simulink model "F3_CAN_LoopBackInterrupt"  (R2018b)
settings: Solver=FixedStepDiscrete  StartTime=0.0  StopTime=10.0  RelTol=1e-3  EnableMultiTasking=on
libraries: CAN_Lib x13, canmsglib x2, STM32_Config_Lib x1
settings Model: Creator=reynaudp  LastModifiedBy=fenard1
settings DataIOCC: LimitDataPoints=on  SaveFormat=Array
settings OptimizationCC: DefaultParameterBehavior=Inlined  DefaultUnderspecifiedDataType=single  PassReuseOutputArgsAs=Individual arguments  LifeSpan=1
settings DebuggingCC: SolverPrmCheckMsg=warning  UniqueDataStoreMsg=error  AllowSymbolicDim=off  StrictBusMsg=ErrorOnBusTreatedAsVector  SFUnexpectedBacktrackingDiag=warning  SFNoUnconditionalDefaultTransitionDiag=warning  SFUndirectedBroadcastEventsDiag=error  SFExecutionAtInitializationDiag=none
settings HardwareCC: ProdBitPerPointer=32  ProdBitPerSizeT=32  ProdBitPerPtrDiffT=32  ProdLargestAtomicInteger=Integer  ProdWordSize=32  ProdHWDeviceType=STMicroelectronics->STM32 32-bit Cortex-M
settings ModelReferenceCC: PropagateSignalLabelsOutOfModel=off
settings SFSimCC: SimUseLocalCustomCode=off  CompileTimeRecursionLimit=0  EnableRuntimeRecursion=off  MATLABDynamicMemAlloc=off
settings RTWCC: SystemTargetFile=stm32.tlc  TemplateMakefile=stm32.tmf  Description=stm32 (Embedded Target)  GenerateReport=on  RTWUseLocalCustomCode=off  Toolchain=Microsoft Windows SDK v7.1 | nmake (64-bit Windows)
settings CodeAppCC: IgnoreCustomStorageClasses=off  CustomSymbolStrType=$N$R$M  SimulinkBlockComments=off
settings STFCustomTargetCC: TargetLangStandard=C99 (ISO)  ParMdlRefBuildCompliant=on  IncludeMdlTerminateFcn=off  CombineOutputUpdateFcns=on  ERTCustomFileBanners=on  SupportComplex=off  SupportContinuousTime=off  SupportNonInlinedSFcns=off  RemoveResetFunc=on  ParenthesesLevel=Maximum  CastingMode=Standards  MATLABClassNameForMDSCustomization=Simulink.SoftwareTarget.ERTCustomization  SystemTargetFile=stm32.tlc
settings ERTTargetCC: TargetLangStandard=C99 (ISO)  MultiwordLength=2048  CompOptLevelCompliant=off  ConcurrentExecutionCompliant=off  IncludeMdlTerminateFcn=off  SupportComplex=off  ParenthesesLevel=Maximum  CastingMode=Standards  ModelStepFunctionPrototypeControlCompliant=off  CPPClassGenCompliant=off  UseToolchainInfoCompliant=off  ERTSrcFileBannerTemplate=sourceFileTemplate.cgt  ERTHdrFileBannerTemplate=sourceFileTemplate.cgt  ERTDataSrcFileTemplate=sourceFileTemplate.cgt  ERTDataHdrFileTemplate=sourceFileTemplate.cgt  ERTCustomFileTemplate=customRoutineProcess.tlc  ConvertIfToSwitch=off  SuppressUnreachableDefaultCases=off  EnableSignedLeftShifts=off  EnableSignedRightShifts=off
settings ConfigComp: CovMetricSettings=dw  CovHtmlReporting=on  CovSaveCumulativeToWorkspaceVar=on  CovSaveSingleToWorkspaceVar=on  CovExternalEMLEnable=off  CovSFcnEnable=off

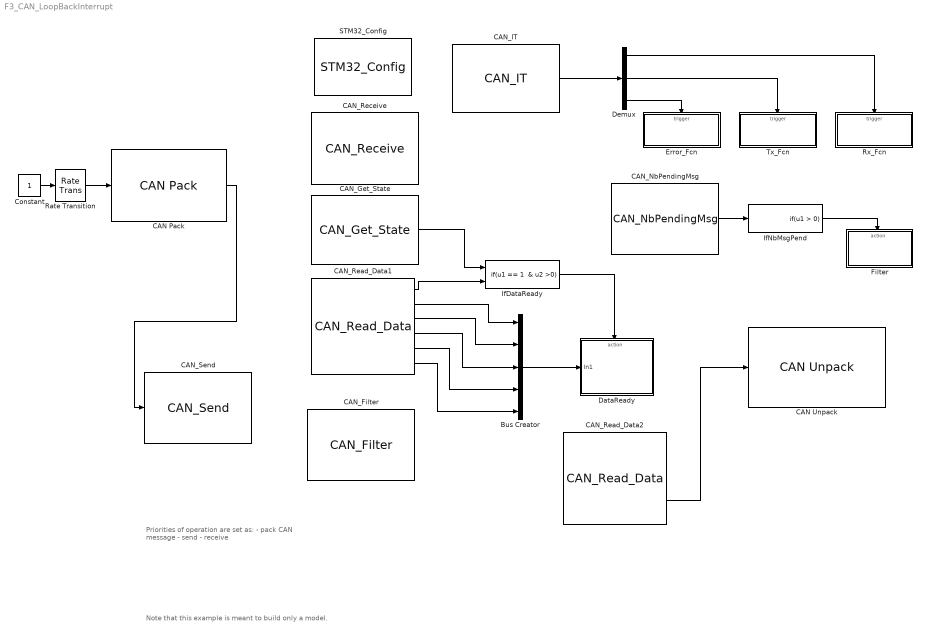
== system F3_CAN_LoopBackInterrupt ==
  note: Priorities of operation are set as:
      | - pack CAN message
      | - send
      | - receive
  note: Note that this example is meant to build only a model.
  Bus Creator : BusCreator  Inputs=5
  CAN Pack : canmsglib/CAN Pack  Priority=1  MsgList=(none)  MsgName=CAN Msg  MsgIDType=Extended (29-bit identifier)  MsgIdentifier=0  MsgLength=8  SignalInfo=Signal1$0$8$1$1$1$0$1$0$-Inf$Inf$#  NSignals=1  StartBits=str2num('[int32(0)]')  SignalSizes=str2num('[int32(8)]')  ByteOrders=str2num('[int32(1)]')  DataTypes=str2num('[int32(1)]')  MultiplexTypes=str2num('[int32(1)]')  MultiplexValues=str2num('[double(0)]')  Factors=str2num('[double(1)]')  Offsets=str2num('[double(0)]')  Minimums=str2num('[double(-Inf)]')  Maximums=str2num('[double(Inf)]')  Remote=off  ApplyMinMax=off  BusOutput=off
      settings: AttributesFormatString=Priority=%<Priority>  SourceProductName=Vehicle Network Toolbox  SourceProductBaseCode=VN  DataFormat=manually specified signals
  CAN Unpack : canmsglib/CAN Unpack  MsgList=(none)  MsgName=CAN Msg  MsgIDType=Standard (11-bit identifier)  MsgIdentifier=0  MsgLength=8  NSignals=0  IDPort=on  TimestampPort=on  ErrorPort=on  RemotePort=on  LengthPort=on  StatusPort=on  StartBits=0  SignalSizes=0  ByteOrders=0  DataTypes=0  MultiplexTypes=0  MultiplexValues=0  Factors=0  Offsets=0  Minimums=0  Maximums=0  ApplyMinMax=off
      settings: SourceProductName=Vehicle Network Toolbox  SourceProductBaseCode=VN  DataFormat=raw data
  CAN_Filter : CAN_Lib/CAN_Filter  CAN_name=CAN  CAN_Filter_Activation=on  CAN_Filter_Scale=CAN_FILTERSCALE_32BIT  CAN_Filter_Mask_Id_High=0  CAN_Filter_Mask_Id_Low=0  CAN_Filter_Id_High=0  CAN_Filter_Id_Low=0  CAN_Filter_FIFO_Assignment=CAN_FIFO0  CAN_Filter_Bank=0  CAN_Filter_Mode=CAN_FILTERMODE_IDMASK  CAN_Filter_Slave_Start_Bank=14
      settings: SourceProductName=Target Support Package - STM32 Adapter
  CAN_Get_State : CAN_Lib/CAN_Get_State  CAN_name=CAN
      settings: SourceProductName=Target Support Package - STM32 Adapter
  CAN_IT : CAN_Lib/CAN_IT  CAN_name=CAN  CAN_Mode=Master  CAN_It=on  CAN_RX_It=on  CAN_TX_It=on  CAN_ERROR_It=on
      settings: SourceProductName=Target Support Package - STM32 Adapter
  CAN_NbPendingMsg : CAN_Lib/CAN_NbPendingMsg  CAN_name=CAN  CAN_Mode=Master  CAN_It=on  CAN_Fifo=CAN_FIFO0
      settings: SourceProductName=Target Support Package - STM32 Adapter
  CAN_Read_Data1 : CAN_Lib/CAN_Read_Data  CAN_name=CAN  CAN_Fifo=CAN_FIFO0  CAN_MsgType=off
      settings: SourceProductName=Target Support Package - STM32 Adapter
  CAN_Read_Data2 : CAN_Lib/CAN_Read_Data  CAN_name=CAN  CAN_Fifo=CAN_FIFO0  CAN_MsgType=on
      settings: SourceProductName=Target Support Package - STM32 Adapter
  CAN_Receive : CAN_Lib/CAN_Receive  Priority=2  CAN_name=CAN  CAN_Mode=Master  CAN_It=on  CAN_Fifo=CAN_FIFO0
      settings: AttributesFormatString=Priority=%<Priority>  SourceProductName=Target Support Package - STM32 Adapter
  CAN_Send : CAN_Lib/CAN_Send  Priority=2  CAN_name=CAN  CAN_Mode=Master  CAN_It=on  CAN_MsgType=on
      settings: AttributesFormatString=Priority=%<Priority>  SourceProductName=Target Support Package - STM32 Adapter
  Constant : Constant
  DataReady : Subsystem  TreatAsAtomicUnit=on
  Demux : Demux  Outputs=3
  Error_Fcn : Subsystem  TreatAsAtomicUnit=on
  Filter : Subsystem  TreatAsAtomicUnit=on
  IfDataReady : If  NumInputs=2  IfExpression="u1 == 1  & u2 >0"  ShowElse=off
  IfNbMsgPend : If  ShowElse=off
  Rate Transition : RateTransition
  Rx_Fcn : Subsystem  TreatAsAtomicUnit=on
  STM32_Config : STM32_Config_Lib/STM32_Config  Priority=0  Project_Path=.\  Config_File=F3_CAN_LoopBackInterrupt.ioc  MCU_Name=STM32F302R8Tx
      settings: SourceProductName=Target Support Package - STM32 Adapter
  Tx_Fcn : Subsystem  TreatAsAtomicUnit=on
  wires:
  CAN_IT/1 -> Demux/1
  Demux/1 -> Rx_Fcn/Trigger
  Demux/2 -> Tx_Fcn/Trigger
  Demux/3 -> Error_Fcn/Trigger
  IfDataReady/1 -> DataReady/Action
  CAN_Read_Data1/2 -> Bus Creator/1
  CAN_Read_Data1/3 -> Bus Creator/2
  CAN_Read_Data1/4 -> Bus Creator/3
  Bus Creator/1 -> DataReady/1(In1)
  CAN_Get_State/1 -> IfDataReady/1
  CAN_NbPendingMsg/1 -> IfNbMsgPend/1
  IfNbMsgPend/1 -> Filter/Action
  CAN_Read_Data1/1 -> IfDataReady/2
  CAN_Read_Data2/2 -> CAN Unpack/1
  CAN_Read_Data1/5 -> Bus Creator/4
  CAN_Read_Data1/6 -> Bus Creator/5
  CAN Pack/1 -> CAN_Send/1
  Constant/1 -> Rate Transition/1
  Rate Transition/1 -> CAN Pack/1

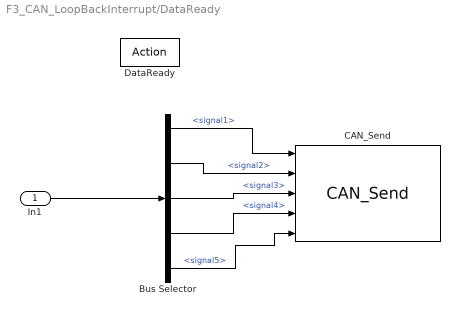
== system F3_CAN_LoopBackInterrupt/DataReady ==
  In1 : Inport
  DataReady : ActionPort  ActionType=then
  Bus Selector : BusSelector  OutputSignals=signal1,signal2,signal3,signal4,signal5
  CAN_Send : CAN_Lib/CAN_Send  CAN_name=CAN  CAN_Mode=Master  CAN_It=on  CAN_MsgType=off
      settings: SourceProductName=Target Support Package - STM32 Adapter
  wires:
  In1/1 -> Bus Selector/1
  Bus Selector/2 -> CAN_Send/2  "<signal2>"
  Bus Selector/3 -> CAN_Send/3  "<signal3>"
  Bus Selector/4 -> CAN_Send/4  "<signal4>"
  Bus Selector/5 -> CAN_Send/5  "<signal5>"
  Bus Selector/1 -> CAN_Send/1  "<signal1>"

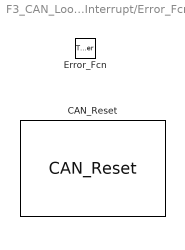
== system F3_CAN_LoopBackInterrupt/Error_Fcn ==
  Error_Fcn : TriggerPort  TriggerType=function-call  VariantControl=Variant
  CAN_Reset : CAN_Lib/CAN_Reset  CAN_name=CAN
      settings: SourceProductName=Target Support Package - STM32 Adapter

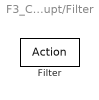
== system F3_CAN_LoopBackInterrupt/Filter ==
  Filter : ActionPort  ActionType=then

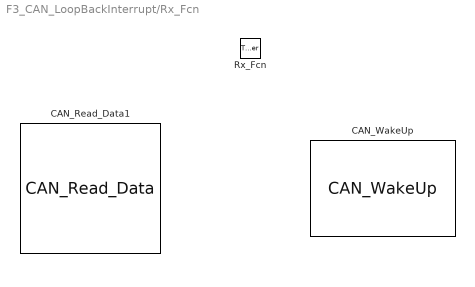
== system F3_CAN_LoopBackInterrupt/Rx_Fcn ==
  Rx_Fcn : TriggerPort  TriggerType=function-call  VariantControl=Variant
  CAN_Read_Data1 : CAN_Lib/CAN_Read_Data  CAN_name=CAN  CAN_Fifo=CAN_FIFO0  CAN_MsgType=off
      settings: SourceProductName=Target Support Package - STM32 Adapter
  CAN_WakeUp : CAN_Lib/CAN_WakeUp  CAN_name=CAN  CAN_Mode=Master  CAN_It=on
      settings: SourceProductName=Target Support Package - STM32 Adapter

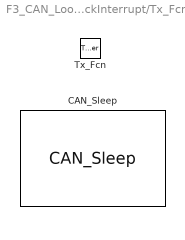
== system F3_CAN_LoopBackInterrupt/Tx_Fcn ==
  Tx_Fcn : TriggerPort  TriggerType=function-call  VariantControl=Variant
  CAN_Sleep : CAN_Lib/CAN_Sleep  CAN_name=CAN  CAN_Mode=Master  CAN_It=on
      settings: SourceProductName=Target Support Package - STM32 Adapter
